simulink library "CommonBlocks"  (R2019a)
settings: Solver=VariableStepAuto  StartTime=0.0  StopTime=10.0  RelTol=1e-3
settings Model: Creator=Peter  LastModifiedBy=jakub

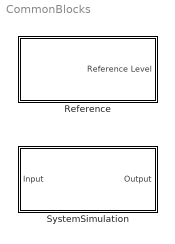
== system CommonBlocks ==
  Reference : Subsystem  mask{RefVect=[65, 50, 35, 45, 60, 75, 55, 40, 20, 30], AtTheEnd=Stop simulation, Reps=5, SectLen=2400, OffsetTime=0, Ts=0.025}
      mask prompts: RefVect "Reference vector:"; AtTheEnd "After reaching end of Reference vector:"; Reps "Total number of Reference vector repetitions (N):"; SectLen "Section length (number of samples):"; OffsetTime "Offset time at start (reserved for calibration etc.) (s):"; Ts "Sampling period (s):"
      mask TypeOptions AtTheEnd: Stop simulation | Start from beginning | Start from beginning N-1 times then stop simulation
      mask Callback AtTheEnd:
      | CurrentBlock = gcb;
      | EndAction = get_param(CurrentBlock,'AtTheEnd');
      | Menu = Simulink.Mask.get(CurrentBlock);
      | RepOpt = Menu.getParameter('Reps');
      | 
      | 
      | if strcmp(EndAction,'Stop simulation')
      | RepOpt.Enabled='off';
      | elseif strcmp(EndAction,'Start from beginning')
      | RepOpt.Enabled='off';
      | else
      | RepOpt.Enabled='on';
      | end
      mask DialogControl DescGroupVar Prompt: Reference Block
      mask DialogControl DescTextVar Prompt: Block used to provide changing reference levels during simulation.
      mask DialogControl Reps Tooltip: Including first repetition, so the value needs to be greater or equal 1.
  SystemSimulation : Subsystem  mask{repre=Transfer function, IC=0, system=0}
      mask prompts: repre "Representation of the system"; IC "Initial conditions"; system "System variable name"
      mask help:
      | This block provides the possibility to simulate a representation of the a particular system.
      | The representation can be in the form of:
      | - Transfer Function (TF)
      | - State-Space Representation (SS)
      | - Discrete State-Space Representation (dSS)
      | In the 'System variable name' field  is the variable representing the system with suficient datatype required (supported datatype: ss, idss, tf).
      mask init:
      | set_param(gcb, 'MaskSelfModifiable', 'on');
      mask TypeOptions repre: Transfer function | State-Space | Discrete State-Space
      mask Callback repre:
      | mask_popup = get_param(gcb,'repre'); % which popup is choosen
      | % path to the representations blocks
      | path = gcb;
      | wayTF = strcat(path,'/Transfer Fcn');
      | waySS = strcat(path,'/State-Space');
      | waydSS = strcat(path,'/Discrete State-Space');
      | % coment out bolcks that are not picked
      | if strcmp(mask_popup(1),'T')
      |     set_param(wayTF,'commented','off');
      |     set_param(waySS,'commented','on');
      |     set_param(waydSS,'commented','on');
      |     set_param(gcb,'MaskVisibilities',{'on','off','on'}); %Initial conditions visibility
      | elseif strcmp(mask_popup(1),'S')
      |     set_param(waySS,'commented','off');
      |     set_param(wayTF,'commented','on');
      |     set_param(waydSS,'commented','on');
      |     set_param(gcb,'MaskVisibilities',{'on','on','on'}); %Initial conditions visibility
      | else
      |     set_param(waydSS,'commented','off');
      |     set_param(waySS,'commented','on');
      |     set_param(wayTF,'commented','on');
      |     set_param(gcb,'MaskVisibilities',{'on','on','on'}); %Initial conditions visibility
      | end
      mask Callback system:
      | % Prevent the situation that windov for system
      | % representation is empty
      | mask_field = get_param(gcb,'system');
      | path = gcb;
      | wayTF = strcat(path,'/Transfer Fcn');
      | waySS = strcat(path,'/State-Space');
      | waydSS = strcat(path,'/Discrete State-Space');
      | if isempty(mask_field)
      |     set_param(gcb,'system','0');
      |     set_param(wayTF,'commented','on');
      |     set_param(waySS,'commented','on');
      |     set_param(waydSS,'commented','on');
      | end
      mask DialogControl DescGroupVar Prompt: SystemSimulation block

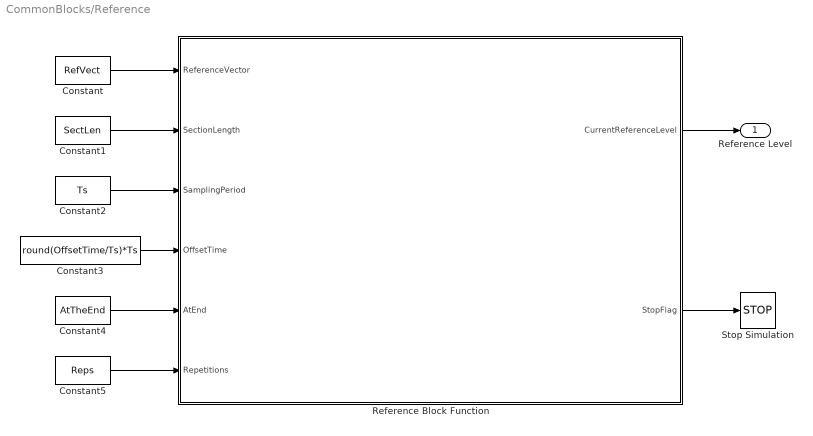
== system CommonBlocks/Reference ==
  Constant : Constant  Value=RefVect  SampleTime=Ts
  Constant1 : Constant  Value=SectLen  SampleTime=Ts
  Constant2 : Constant  Value=Ts  SampleTime=Ts
  Constant3 : Constant  Value=round(OffsetTime/Ts)*Ts  SampleTime=Ts
  Constant4 : Constant  Value=AtTheEnd  SampleTime=Ts
  Constant5 : Constant  Value=Reps  SampleTime=Ts
  Reference Block Function : MATLAB Function  TreatAsAtomicUnit=on
  Stop Simulation : Stop
  Reference Level : Outport
  wires:
  Constant/1 -> Reference Block Function/1(ReferenceVector)
  Constant1/1 -> Reference Block Function/2(SectionLength)
  Constant2/1 -> Reference Block Function/3(SamplingPeriod)
  Constant3/1 -> Reference Block Function/4(OffsetTime)
  Reference Block Function/1(CurrentReferenceLevel) -> Reference Level/1
  Reference Block Function/2(StopFlag) -> Stop Simulation/1
  Constant4/1 -> Reference Block Function/5(AtEnd)
  Constant5/1 -> Reference Block Function/6(Repetitions)

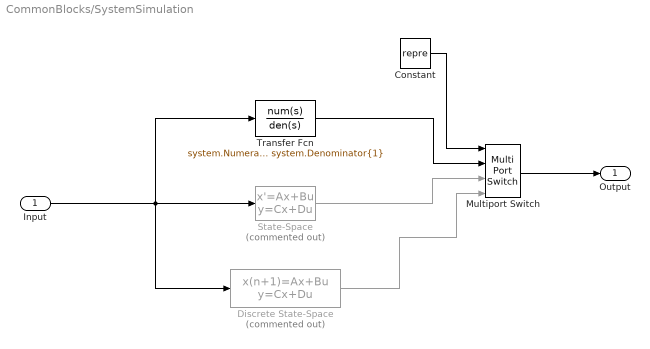
== system CommonBlocks/SystemSimulation ==
  Input : Inport
  Constant : Constant  Value=repre
  Discrete State-Space : DiscreteStateSpace  Commented=on  A=system.A  B=system.B  C=system.C  D=system.D  InitialCondition=IC  SampleTime=system.Ts
  Multiport Switch : MultiPortSwitch
  State-Space : StateSpace  Commented=on  A=system.A  B=system.B  C=system.C  D=system.D  InitialCondition=IC
  Transfer Fcn : TransferFcn  Numerator=system.Numerator{1}  Denominator=system.Denominator{1}
  Output : Outport
  wires:
  Input/1 -> Discrete State-Space/1, State-Space/1, Transfer Fcn/1
  Multiport Switch/1 -> Output/1
  Constant/1 -> Multiport Switch/1
  Discrete State-Space/1 -> Multiport Switch/4
  State-Space/1 -> Multiport Switch/3
  Transfer Fcn/1 -> Multiport Switch/2

== matlab function CommonBlocks/Reference/Reference Block Function ==
  data: CurrentReferenceLevel output; ReferenceVector input; SectionLength input; SamplingPeriod input; StopFlag output; OffsetTime input; AtEnd input; Repetitions input
%     Simulink Block for changing reference train used in PID examples.
%
%     This code is part of the AutomationShield hardware and software
%     ecosystem. Visit http://www.automationshield.com for more
%     details. This code is licensed under a Creative Commons
%     Attribution-NonCommercial 4.0 International License.
%
%     Created by Peter Chmurciak.
%     Last update: 14.8.2019.

function [CurrentReferenceLevel, StopFlag] = fcn(ReferenceVector, SectionLength, SamplingPeriod, OffsetTime, AtEnd, Repetitions)

persistent positionCounter sampleCounter repetitionCounter;       % Persistent variables

if isempty(positionCounter)                                       % Initialisation of persistent variables
    positionCounter = 1;                                          % Counter for current position in reference train 
    sampleCounter = 0;                                            % Counter for number of samples in section
    repetitionCounter = 0;                                        % Counter for number of repetitions of reference train
end

if repetitionCounter == 0 && positionCounter == 1                      % First run
    CurrentReferenceLevel = ReferenceVector(positionCounter);
    sampleCounter = sampleCounter + 1;
    StopFlag = 0;
    if sampleCounter == (SectionLength + OffsetTime / SamplingPeriod)  % Implement offset for calibration etc.
        positionCounter = positionCounter + 1;
        sampleCounter = 0;
    end
elseif positionCounter < length(ReferenceVector)                       % Changing reference train
    CurrentReferenceLevel = ReferenceVector(positionCounter);
    sampleCounter = sampleCounter + 1;
    StopFlag = 0;
    if sampleCounter == SectionLength
        positionCounter = positionCounter + 1;                         % Move further in reference
        sampleCounter = 0;
    end
else
    CurrentReferenceLevel = ReferenceVector(positionCounter);
    sampleCounter = sampleCounter + 1;
    if sampleCounter == SectionLength
        if AtEnd == 1                                                  % Decision based on mode selected by user
            StopFlag = 1;                                              % Stop simulation at the end of reference train
        elseif AtEnd == 2
            StopFlag = 0;
            positionCounter = 1;                                       % Start reference train from the beginning
            sampleCounter = 0;
            repetitionCounter = repetitionCounter + 1;                 % Increment repetition counter
        else
            positionCounter = 1;                                       % Start reference train from the beginning
            sampleCounter = 0;
            repetitionCounter = repetitionCounter + 1;                 % Increment repetition counter
            if repetitionCounter == Repetitions
                StopFlag = 1;                                          % Stop simulation if train was repeated N times
            else
                StopFlag = 0;
            end
        end
    else
        StopFlag = 0;
    end
end

end   % End of function definition
